simulink subsystem "passive_balancing_logic"  (R2021a)
settings: Solver=VariableStepAuto  StartTime=0.0  StopTime=10.0  RelTol=1e-3
settings Model: Creator=Carlo Edoardo  LastModifiedBy=Carlo Edoardo

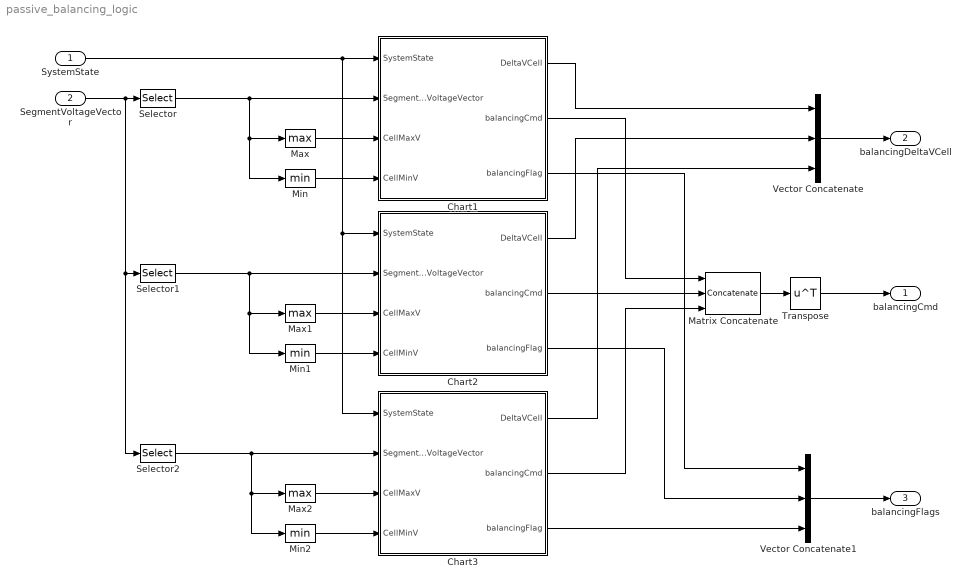
== system passive_balancing_logic ==
  SystemState : Inport  OutDataTypeStr=Enum: SystemState_t
  SegmentVoltageVector : Inport  Port=2
  Chart1 : Stateflow chart  TreatAsAtomicUnit=on
      settings: PortSchema="{\"entries\":[{\"content\":{\"sides\":[{\"content\":{\"connectorIds\":[\"In1\",\"In2\",\"In3\",\"In4\"]},\"type\":\"ConnectorPlacement.EquallySpacedRectSide\",\"uuid\":\"a2741edf-0a6a-4cdc-8864-68b68dbb5e7b\"},{\"content\":{\"connectorIds\":[\"Out2\",\"Out1\",\"Out3\"],\"side\":\"RIGHT\"},\"type\":\"ConnectorPlacement.EquallySpacedRectSide\",\"uuid\":\"3e33edf4-8d09-490e-8b71-f55d7866ff69\"},{\"content\":{\"connectorIds\":[],\"side\":\"TOP\"},\"type\":\"ConnectorPlacement.EquallySpacedRectSide\",\"uuid\":\"52eb0d7a-a4df-4df7-91e4-464aa4e0ab31\"}]},\"type\":\"ConnectorPlacement.EquallySpacedConnector\",\"uuid\":\"8927709b-3b25-412c-93a6-8f62d2d50716\"}],\"packageUris\":[\"http://schema.mathworks.com/mf0/Connector/R2020b\"],\"version\":\"1.0\"}"
  Chart2 : Stateflow chart  TreatAsAtomicUnit=on
      settings: PortSchema="{\"entries\":[{\"content\":{\"sides\":[{\"content\":{\"connectorIds\":[\"In1\",\"In2\",\"In3\",\"In4\"]},\"type\":\"ConnectorPlacement.EquallySpacedRectSide\",\"uuid\":\"a2741edf-0a6a-4cdc-8864-68b68dbb5e7b\"},{\"content\":{\"connectorIds\":[\"Out2\",\"Out1\",\"Out3\"],\"side\":\"RIGHT\"},\"type\":\"ConnectorPlacement.EquallySpacedRectSide\",\"uuid\":\"3e33edf4-8d09-490e-8b71-f55d7866ff69\"},{\"content\":{\"connectorIds\":[],\"side\":\"TOP\"},\"type\":\"ConnectorPlacement.EquallySpacedRectSide\",\"uuid\":\"52eb0d7a-a4df-4df7-91e4-464aa4e0ab31\"}]},\"type\":\"ConnectorPlacement.EquallySpacedConnector\",\"uuid\":\"8927709b-3b25-412c-93a6-8f62d2d50716\"}],\"packageUris\":[\"http://schema.mathworks.com/mf0/Connector/R2020b\"],\"version\":\"1.0\"}"
  Chart3 : Stateflow chart  TreatAsAtomicUnit=on
      settings: PortSchema="{\"entries\":[{\"content\":{\"sides\":[{\"content\":{\"connectorIds\":[\"In1\",\"In2\",\"In3\",\"In4\"]},\"type\":\"ConnectorPlacement.EquallySpacedRectSide\",\"uuid\":\"a2741edf-0a6a-4cdc-8864-68b68dbb5e7b\"},{\"content\":{\"connectorIds\":[\"Out2\",\"Out1\",\"Out3\"],\"side\":\"RIGHT\"},\"type\":\"ConnectorPlacement.EquallySpacedRectSide\",\"uuid\":\"3e33edf4-8d09-490e-8b71-f55d7866ff69\"},{\"content\":{\"connectorIds\":[],\"side\":\"TOP\"},\"type\":\"ConnectorPlacement.EquallySpacedRectSide\",\"uuid\":\"52eb0d7a-a4df-4df7-91e4-464aa4e0ab31\"}]},\"type\":\"ConnectorPlacement.EquallySpacedConnector\",\"uuid\":\"8927709b-3b25-412c-93a6-8f62d2d50716\"}],\"packageUris\":[\"http://schema.mathworks.com/mf0/Connector/R2020b\"],\"version\":\"1.0\"}"
  Matrix Concatenate : Concatenate  NumInputs=3  Mode=Multidimensional array  ConcatenateDimension=2
  Max : MinMax  Function=max
  Max1 : MinMax  Function=max
  Max2 : MinMax  Function=max
  Min : MinMax
  Min1 : MinMax
  Min2 : MinMax
  Selector : Selector  NumberOfDimensions=2  InputPortWidth=3  IndexOptions=Starting index (dialog),Select all  Indices=1,1  OutputSizes=1,1
  Selector1 : Selector  NumberOfDimensions=2  InputPortWidth=3  IndexOptions=Starting index (dialog),Select all  Indices=1,1  OutputSizes=1,1
  Selector2 : Selector  NumberOfDimensions=2  InputPortWidth=3  IndexOptions=Starting index (dialog),Select all  Indices=1,1  OutputSizes=1,1
  Transpose : Math  Operator=transpose  SaturateOnIntegerOverflow=on
  Vector Concatenate : Concatenate  NumInputs=3
  Vector Concatenate1 : Concatenate  NumInputs=3
  balancingCmd : Outport
  balancingDeltaVCell : Outport  Port=2
  balancingFlags : Outport  Port=3
  wires:
  Max/1 -> Chart1/3(CellMaxV)
  SystemState/1 -> Chart2/1(SystemState), Chart3/1(SystemState), Chart1/1(SystemState)
  SegmentVoltageVector/1 -> Selector/1, Selector1/1, Selector2/1
  Selector/1 -> Max/1, Min/1, Chart1/2(SegmentVoltageVector)
  Max1/1 -> Chart2/3(CellMaxV)
  Selector1/1 -> Max1/1, Min1/1, Chart2/2(SegmentVoltageVector)
  Max2/1 -> Chart3/3(CellMaxV)
  Selector2/1 -> Max2/1, Min2/1, Chart3/2(SegmentVoltageVector)
  Min2/1 -> Chart3/4(CellMinV)
  Matrix Concatenate/1 -> Transpose/1
  Min/1 -> Chart1/4(CellMinV)
  Min1/1 -> Chart2/4(CellMinV)
  Transpose/1 -> balancingCmd/1
  Chart1/1(balancingCmd) -> Matrix Concatenate/1
  Chart3/1(balancingCmd) -> Matrix Concatenate/3
  Chart2/1(balancingCmd) -> Matrix Concatenate/2
  Chart1/2(DeltaVCell) -> Vector Concatenate/1
  Chart2/2(DeltaVCell) -> Vector Concatenate/2
  Chart3/2(DeltaVCell) -> Vector Concatenate/3
  Chart1/3(balancingFlag) -> Vector Concatenate1/1
  Chart2/3(balancingFlag) -> Vector Concatenate1/2
  Chart3/3(balancingFlag) -> Vector Concatenate1/3
  Vector Concatenate/1 -> balancingDeltaVCell/1
  Vector Concatenate1/1 -> balancingFlags/1

== stateflow chart passive_balancing_logic/Chart1 ==
  state OFF
    en:
    balancingCmd(:)=0;
    balancingFlag=false;
    en,du:
    DeltaVCell = CellMaxV - CellMinV;
  state ON
    en:balancingFlag=true;
    state WaitRelaxation
      en: balancingCmd(:)=0;
    state Balancing
      en, du:
      balancingCmd = ((SegmentVoltageVector - CellMinV) > DeltaVTargetMin);
      flagBalancingDone=all(~balancingCmd)
    state MeasureVoltages
      DeltaVCell=CellMaxV-CellMinV;
    state BalancingFinished
      en,du:DeltaVCell=CellMaxV-CellMinV;
      balancingFlag=false;
    (default) -> Balancing
    Balancing -> WaitRelaxation [order 2] : [(flagBalancingDone==0)&&...
        | after(800,msec)]
    MeasureVoltages -> Balancing
    Balancing -> BalancingFinished [order 1] : [flagBalancingDone  ==  1]
    BalancingFinished -> Balancing : [DeltaVCell > DeltaVTargetMin]
    WaitRelaxation -> MeasureVoltages : [after(1000,msec)]
  (default) -> OFF
  ON -> OFF : [SystemState  ~=  Balancing]
  OFF -> ON : [(SystemState==Balancing) && ...
      | DeltaVCell > DeltaVTargetMin]
  data: SystemState input Enum: SystemState_t; SegmentVoltageVector input size=10; DeltaVTargetMin parameter; balancingCmd output; CellMaxV input; CellMinV input; flagBalancingDone local; DeltaVCell output; balancingFlag output

== stateflow chart passive_balancing_logic/Chart2 ==
  state OFF
    en:
    balancingCmd(:)=0;
    balancingFlag=false;
    en,du:
    DeltaVCell = CellMaxV - CellMinV;
  state ON
    en:balancingFlag=true;
    state WaitRelaxation
      en: balancingCmd(:)=0;
    state Balancing
      en, du:
      balancingCmd = ((SegmentVoltageVector - CellMinV) > DeltaVTargetMin);
      flagBalancingDone=all(~balancingCmd)
    state MeasureVoltages
      DeltaVCell=CellMaxV-CellMinV;
    state BalancingFinished
      en,du:DeltaVCell=CellMaxV-CellMinV;
      balancingFlag=false;
    (default) -> Balancing
    Balancing -> WaitRelaxation [order 2] : [(flagBalancingDone==0)&&...
        | after(800,msec)]
    MeasureVoltages -> Balancing
    Balancing -> BalancingFinished [order 1] : [flagBalancingDone  ==  1]
    BalancingFinished -> Balancing : [DeltaVCell > DeltaVTargetMin]
    WaitRelaxation -> MeasureVoltages : [after(1000,msec)]
  (default) -> OFF
  ON -> OFF : [SystemState  ~=  Balancing]
  OFF -> ON : [(SystemState==Balancing) && ...
      | DeltaVCell > DeltaVTargetMin]
  data: SystemState input Enum: SystemState_t; SegmentVoltageVector input size=10; DeltaVTargetMin parameter; balancingCmd output; CellMaxV input; CellMinV input; flagBalancingDone local; DeltaVCell output; balancingFlag output

== stateflow chart passive_balancing_logic/Chart3 ==
  state OFF
    en:
    balancingCmd(:)=0;
    balancingFlag=false;
    en,du:
    DeltaVCell = CellMaxV - CellMinV;
  state ON
    en:balancingFlag=true;
    state WaitRelaxation
      en: balancingCmd(:)=0;
    state Balancing
      en, du:
      balancingCmd = ((SegmentVoltageVector - CellMinV) > DeltaVTargetMin);
      flagBalancingDone=all(~balancingCmd)
    state MeasureVoltages
      DeltaVCell=CellMaxV-CellMinV;
    state BalancingFinished
      en,du:DeltaVCell=CellMaxV-CellMinV;
      balancingFlag=false;
    (default) -> Balancing
    Balancing -> WaitRelaxation [order 2] : [(flagBalancingDone==0)&&...
        | after(800,msec)]
    MeasureVoltages -> Balancing
    Balancing -> BalancingFinished [order 1] : [flagBalancingDone  ==  1]
    BalancingFinished -> Balancing : [DeltaVCell > DeltaVTargetMin]
    WaitRelaxation -> MeasureVoltages : [after(1000,msec)]
  (default) -> OFF
  ON -> OFF : [SystemState  ~=  Balancing]
  OFF -> ON : [(SystemState==Balancing) && ...
      | DeltaVCell > DeltaVTargetMin]
  data: SystemState input Enum: SystemState_t; SegmentVoltageVector input size=10; DeltaVTargetMin parameter; balancingCmd output; CellMaxV input; CellMinV input; flagBalancingDone local; DeltaVCell output; balancingFlag output
